simulink model "ProgettoControlliTracciaB1GruppoAIPunto5"  (R2022b)
settings: Solver=VariableStepAuto  StartTime=0.0  StopTime=10.000000  RelTol=1e-3
values from neighbouring files (symbols this model uses):
  u_e = 0    [ProgettoControlliTracciaB1GruppoAI.m]
  y_e = x_2e    (= 100)    [ProgettoControlliTracciaB1GruppoAI.m]
libraries: cstblocks x2
settings Model: Creator=Alessio Benenati  LastModifiedBy=Alessio Benenati

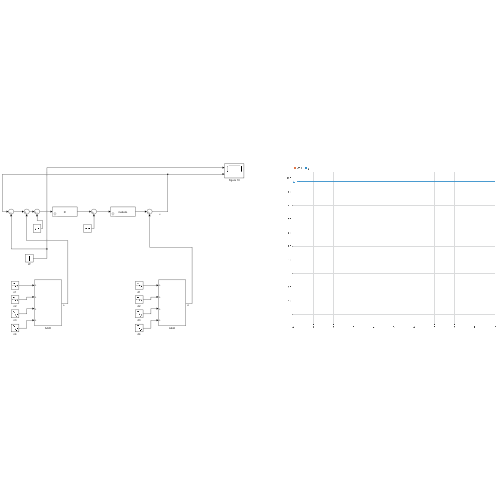
[thumbnail: Simulink's stored preview of the top-level diagram]
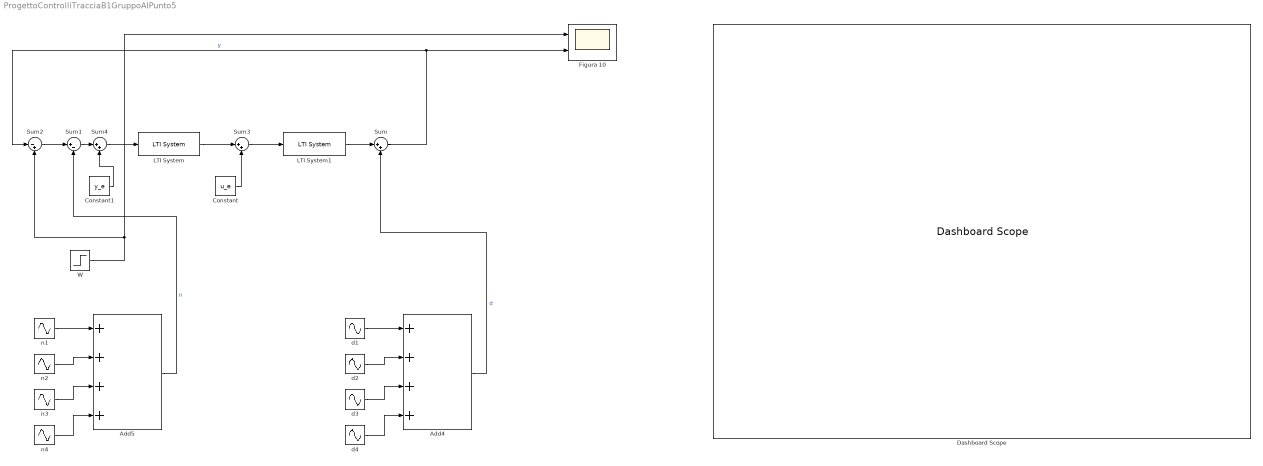
== system ProgettoControlliTracciaB1GruppoAIPunto5 ==
  Add4 : Sum  Inputs=++++
  Add5 : Sum  Inputs=++++
  Constant : Constant  Value=u_e
  Constant1 : Constant  Value=y_e
  Dashboard Scope : DashboardScope
  Figura 10 : Scope  NumInputPorts=2
  LTI System : cstblocks/LTI System  sys=R  IC=[]
  LTI System1 : cstblocks/LTI System  sys=modello  IC=[100,100]
  Sum : Sum  Inputs=|++
  Sum1 : Sum  Inputs=|+-
  Sum2 : Sum  Inputs=|-+
  Sum3 : Sum  Inputs=|++
  Sum4 : Sum  Inputs=|++
  W : Step  Time=0  After=-2  SampleTime=0
  d1 : Sin  Amplitude=0.3  Frequency=0.0125*1  SampleTime=0
  d2 : Sin  Amplitude=0.3  Frequency=0.0125*2  SampleTime=0
  d3 : Sin  Amplitude=0.3  Frequency=0.0125*3  SampleTime=0
  d4 : Sin  Amplitude=0.3  Frequency=0.0125*4  SampleTime=0
  n1 : Sin  Amplitude=0.2  Frequency=10000*1  SampleTime=0
  n2 : Sin  Amplitude=0.2  Frequency=10000*2  SampleTime=0
  n3 : Sin  Amplitude=0.2  Frequency=10000*3  SampleTime=0
  n4 : Sin  Amplitude=0.2  Frequency=10000*4  SampleTime=0
  wires:
  LTI System1/1 -> Sum/1
  W/1 -> Sum2/2, Figura 10/1
  Sum2/1 -> Sum1/1
  Sum1/1 -> Sum4/1
  LTI System/1 -> Sum3/1
  Sum3/1 -> LTI System1/1
  Sum4/1 -> LTI System/1
  d1/1 -> Add4/1
  n1/1 -> Add5/1
  d2/1 -> Add4/2
  d3/1 -> Add4/3
  d4/1 -> Add4/4
  n2/1 -> Add5/2
  n3/1 -> Add5/3
  n4/1 -> Add5/4
  Constant/1 -> Sum3/2
  Add5/1 -> Sum1/2  "n"
  Add4/1 -> Sum/2  "d"
  Sum/1 -> Sum2/1, Figura 10/2  "y"
  Constant1/1 -> Sum4/2
